simulink model "EV_Converter_Model_2"  (R2022b)
settings: Solver=VariableStepAuto  StartTime=0.0  StopTime=10.0  RelTol=1e-3
settings Model: Creator=zs  LastModifiedBy=zs

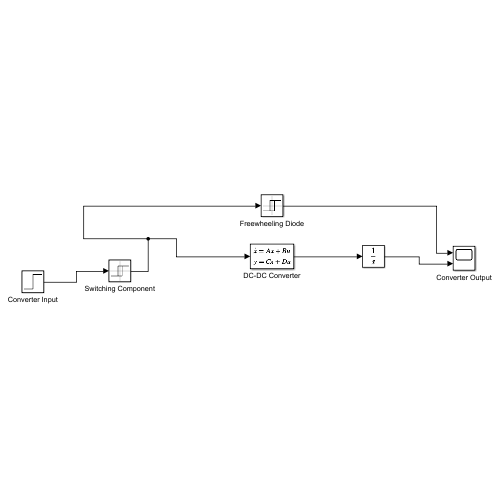
[thumbnail: Simulink's stored preview of the top-level diagram]
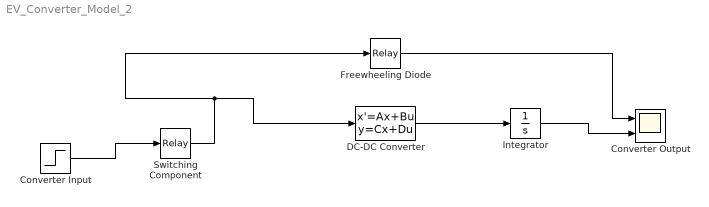
== system EV_Converter_Model_2 ==
  Converter Input : Step  SampleTime=0
  Converter Output : Scope  NumInputPorts=2
  DC-DC Converter : StateSpace  InitialCondition=0
  Freewheeling Diode : Relay
  Integrator : Integrator
  Switching Component : Relay
  wires:
  Converter Input/1 -> Switching Component/1
  Switching Component/1 -> Freewheeling Diode/1, DC-DC Converter/1
  DC-DC Converter/1 -> Integrator/1
  Integrator/1 -> Converter Output/2
  Freewheeling Diode/1 -> Converter Output/1
